simulink model "pendulo_linear_kalman"  (R2020b)
settings: Solver=FixedStepAuto  StartTime=0.0  StopTime=15  FixedStep=1e-3  RelTol=1e-3
values from neighbouring files (symbols this model uses):
  controlador = projetarControlador(requisitos, planta)    [executarTudo.m]    (also in runAll.m = projetarControladorPV(requisitos, planta))
  planta = obterPlanta()    [codetest.m]    (also in executarTudo.m; nextState.m; runAll.m)
  thetar = 0    [executarTudo.m]    (also in runAll.m)
  varCom = 0.01    [runAll.m]
  varMed = 0.001    [runAll.m]
libraries: pid_lib x1
settings Model: Creator=davi  LastModifiedBy=alexandremaranhao

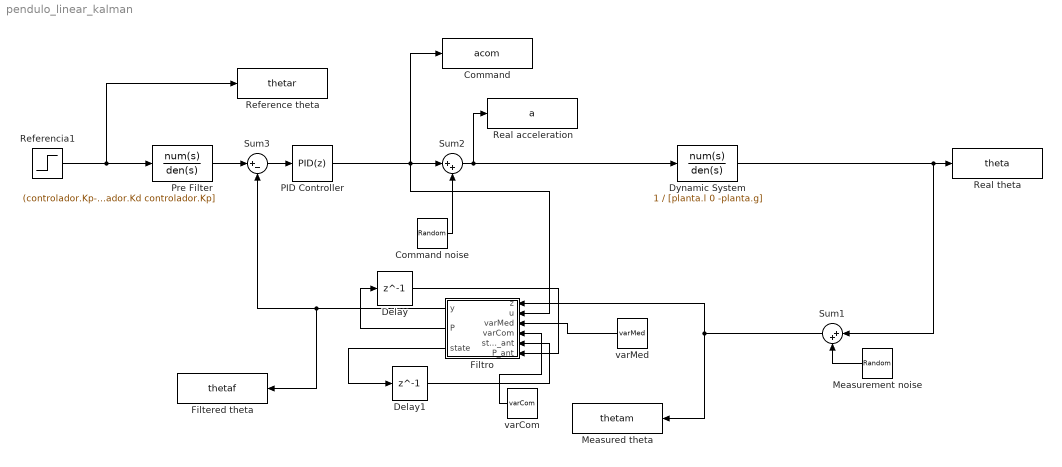
== system pendulo_linear_kalman ==
  Command : ToWorkspace  VariableName=acom  SaveFormat=Structure With Time  SampleTime=-1
  Command noise : RandomNumber  Variance=varCom  SampleTime=0.1
  Delay : Delay  DelayLength=1  InitialCondition=eye(2)  SampleTime=1e-2
  Delay1 : Delay  DelayLength=1  InitialCondition=[0;0]  SampleTime=1e-2
  Dynamic System : TransferFcn  Numerator=1  Denominator=[planta.l 0 -planta.g]
  Filtered theta : ToWorkspace  VariableName=thetaf  SaveFormat=Structure With Time  SampleTime=-1
  Filtro : MATLAB Function  TreatAsAtomicUnit=on  SystemSampleTime=1e-2
  Measured theta : ToWorkspace  VariableName=thetam  SaveFormat=Structure With Time  SampleTime=-1
  Measurement noise : RandomNumber  Variance=varMed  SampleTime=0.1
  PID Controller : pid_lib/PID Controller  Controller=PID  Form=Parallel  TimeDomain=Discrete-time  UseExternalTs=off  SampleTime=1e-2  IntegratorMethod=Forward Euler  FilterMethod=Forward Euler  ControllerParametersSource=internal  P=controlador.Kp  I=0  D=controlador.Kd  UseFilter=on  N=100  TunerSelectOption=Transfer Function Based (PID Tuner App)  InitialConditionSource=internal  InitialConditionForIntegrator=0  InitialConditionForFilter=0  DifferentiatorICPrevScaledInput=0  ExternalReset=none  TrackingMode=off  Kt=1  LimitOutput=off  SatLimitsSource=internal  UpperSaturationLimit=inf  LowerSaturationLimit=-inf  LinearizeAsGain=on  AntiWindupMode=none  Kb=1  POutMin=[]  POutMax=[]  IOutMin=[]  IOutMax=[]  DOutMin=[]  DOutMax=[]  NOutMin=[]  NOutMax=[]  SumOutMin=[]  SumOutMax=[]  SaturationOutMin=[]  SaturationOutMax=[]  PParamMin=[]  PParamMax=[]  IParamMin=[]  IParamMax=[]  DParamMin=[]  DParamMax=[]  NParamMin=[]  NParamMax=[]  KbParamMin=[]  KbParamMax=[]  KtParamMin=[]  KtParamMax=[]  KbOutMin=[]  KbOutMax=[]  KtOutMin=[]  KtOutMax=[]  IntegratorOutMin=[]  IntegratorOutMax=[]  FilterOutMin=[]  FilterOutMax=[]  SumI1OutMin=[]  SumI1OutMax=[]  SumI2OutMin=[]  SumI2OutMax=[]  SumI3OutMin=[]  SumI3OutMax=[]  SumI4OutMin=[]  SumI4OutMax=[]  SumDOutMin=[]  SumDOutMax=[]  DifferentiatorOutMin=[]  DifferentiatorOutMax=[]  FilterDiffOutCoefMin=[]  FilterDiffOutCoefMax=[]  ReciprocalOutMin=[]  ReciprocalOutMax=[]  SumDenOutMin=[]  SumDenOutMax=[]  SumNumOutMin=[]  SumNumOutMax=[]  DivideOutMin=[]  DivideOutMax=[]  UdiffTsProdOutMin=[]  UdiffTsProdOutMax=[]  NTsProdOutMin=[]  NTsProdOutMax=[]  UintegralTsProdOutMin=[]  UintegralTsProdOutMax=[]  UngainTsProdOutMin=[]  UngainTsProdOutMax=[]  IntegratorContinuousStateAttributes=''  IntegratorStateMustResolveToSignalObject=off  IntegratorRTWStateStorageClass=Auto  FilterContinuousStateAttributes=''  FilterStateMustResolveToSignalObject=off  FilterRTWStateStorageClass=Auto  ParallelPVariant=InternalParameters  IdealPVariant=Disabled  IVariant=InternalParameters  DVariant=InternalParameters  IntegratorVariant=Discrete  SatVariant=Disabled  AWVariant=Passthrough  PCopyVariant=Disabled  TRVariant=Disabled  FdbkBlocksVariant=Forward  IdealPFdbkVariant=Disabled  SatFdbkVariant=Disabled  DerivativeFilterVariant=ForwardEulerFilter  NVariant=InternalParameters  NCopyVariant=Disabled  FilterICVariant=InternalICsFilter  IntegratorICVariant=InternalICs  ExternalResetVariant=Disabled  TRSumVariant=Passthrough  SumFdbkVariant=Disabled  SumVariant=Sum_PID  TsampFilterVariant=InternalTs  TsampNgainVariant=Passthrough  TsampIntegralVariant=Passthrough  ExternalSaturationOutDataTypeStr=Inherit: Same as second input
  Pre Filter : TransferFcn  Numerator=(controlador.Kp-planta.g)/planta.l  Denominator=[controlador.Kd controlador.Kp]
  Real acceleration : ToWorkspace  VariableName=a  SaveFormat=Structure With Time  SampleTime=-1
  Real theta : ToWorkspace  VariableName=theta  SaveFormat=Structure With Time  SampleTime=-1
  Reference theta : ToWorkspace  VariableName=thetar  SaveFormat=Structure With Time  SampleTime=-1
  Referencia1 : Step  Time=0  After=thetar  SampleTime=0
  Sum1 : Sum  Inputs=|++
  Sum2 : Sum  Inputs=|++
  Sum3 : Sum  Inputs=|+-
  varCom : Constant  Value=varCom
  varMed : Constant  Value=varMed
  wires:
  Measurement noise/1 -> Sum1/2
  Sum2/1 -> Real acceleration/1, Dynamic System/1
  Command noise/1 -> Sum2/2
  Referencia1/1 -> Pre Filter/1, Reference theta/1
  Pre Filter/1 -> Sum3/1
  Dynamic System/1 -> Real theta/1, Sum1/1
  Sum3/1 -> PID Controller/1
  varMed/1 -> Filtro/3(varMed)
  varCom/1 -> Filtro/4(varCom)
  PID Controller/1 -> Filtro/2(u), Command/1, Sum2/1
  Sum1/1 -> Measured theta/1, Filtro/1(z)
  Filtro/1(y) -> Filtered theta/1, Sum3/2
  Filtro/3(state) -> Delay1/1
  Filtro/2(P) -> Delay/1
  Delay1/1 -> Filtro/5(state_ant)
  Delay/1 -> Filtro/6(P_ant)

== matlab function pendulo_linear_kalman/Filtro ==
  settings: updateMethod=DISCRETE
  data: z input; y output; u input; varMed input; varCom input; state_ant input; P_ant input; P output; state output
function [y,P, state] = fcn(z, u, varMed, varCom, state_ant, P_ant)

F = [1.0010    0.0100; 0.1963    1.0010];
G = [0.0001; 0.02];
n=2;
Q=varCom*eye(n); %covariance of process
R=varMed;        %covariance of measurement  

x_pred = F*state_ant + G*u;
P_pred = F*P_ant*F' + Q;

C = [1 0];
Kt = P_pred * C' * pinv(R + C*P_pred*C');
state = x_pred + Kt*(z-C*state_ant);
P = P_pred - Kt*C*P_pred;
y = state(1);
% y = z;
% P=eye(2);
% state = [0; 0];
end
